simulink model "pendcart"  (R2015b)
settings: Solver=ode45  StartTime=0.0  StopTime=tsim  RelTol=1e-3
values from neighbouring files (symbols this model uses):
  b = 0.01    [old.m]
  c = 0.05    [old.m]
  g = 9.82    [old.m]
  K1 = -119.0071    [old.m]
  K2 = 0.0402    [old.m]
  l = 0.5    [old.m]
  M = 1    [old.m]
  m = 0.5    [old.m]
  p = 5.4277    [old.m]
  p1 = 25.4277    [old.m]
  theta0 = 5*pi/180    (= 0.0872664625997)    [old.m]
settings Model: Creator=Chris  LastModifiedBy=C3204612
settings DataIOCC: SaveFormat=Array  SignalLoggingSaveFormat=ModelDataLogs
settings OptimizationCC: ExpressionDepthLimit=2147483647  InitFltsAndDblsToZero=on
settings DebuggingCC: AlgebraicLoopMsg=none  SaveWithParameterizedLinksMsg=none  UnderspecifiedInitializationDetection=Classic  MergeDetectMultiDrivingBlocksExec=none  FcnCallInpInsideContextMsg=UseLocalSettings  StateNameClashWarn=warning
settings HardwareCC: ProdBitPerPointer=32  ProdLargestAtomicFloat=None  ProdIntDivRoundTo=Undefined  ProdEndianess=Unspecified  ProdWordSize=32  ProdHWDeviceType=32-bit Generic
settings GRTTargetCC: TargetFcnLib=ansi_tfl_tmw.mat  GeneratePreprocessorConditionals=Disable all  CombineOutputUpdateFcns=off  GRTInterface=on
settings ConfigComp: CovModelRefEnable=Off

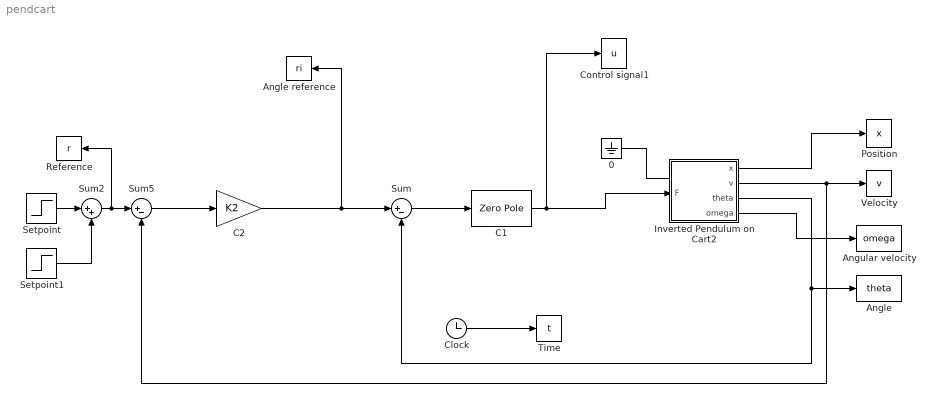
== system pendcart ==
  0 : Ground
  Angle : ToWorkspace  VariableName=theta  SampleTime=-1
  Angle reference : ToWorkspace  VariableName=ri  SampleTime=-1
  Angular velocity : ToWorkspace  VariableName=omega  SampleTime=-1
  C1 : ZeroPole  Zeros=[-p]  Poles=[-p1]  Gain=[K1]
  C2 : Gain  Gain=K2
  Clock : Clock
  Control signal1 : ToWorkspace  VariableName=u  SampleTime=-1
  Inverted Pendulum on Cart2 : Subsystem
  Position : ToWorkspace  VariableName=x  SampleTime=-1
  Reference : ToWorkspace  VariableName=r  SampleTime=-1
  Setpoint : Step  Time=10  After=0.5  SampleTime=0
  Setpoint1 : Step  Time=20  After=-0.5  SampleTime=0
  Sum : Sum  Inputs=|+-
  Sum2 : Sum  Inputs=|++
  Sum5 : Sum  Inputs=|+-
  Time : ToWorkspace  VariableName=t  SampleTime=-1
  Velocity : ToWorkspace  VariableName=v  SampleTime=-1
  wires:
  Clock/1 -> Time/1
  Inverted Pendulum on Cart2/1(x) -> Position/1
  Sum/1 -> C1/1
  C1/1 -> Control signal1/1, Inverted Pendulum on Cart2/1(F)
  Inverted Pendulum on Cart2/4(omega) -> Angular velocity/1
  Inverted Pendulum on Cart2/2(v) -> Velocity/1, Sum5/2
  Inverted Pendulum on Cart2/3(theta) -> Angle/1, Sum/2
  Sum5/1 -> C2/1
  C2/1 -> Angle reference/1, Sum/1
  Setpoint/1 -> Sum2/1
  Setpoint1/1 -> Sum2/2
  Sum2/1 -> Sum5/1, Reference/1
  0/1 -> ?

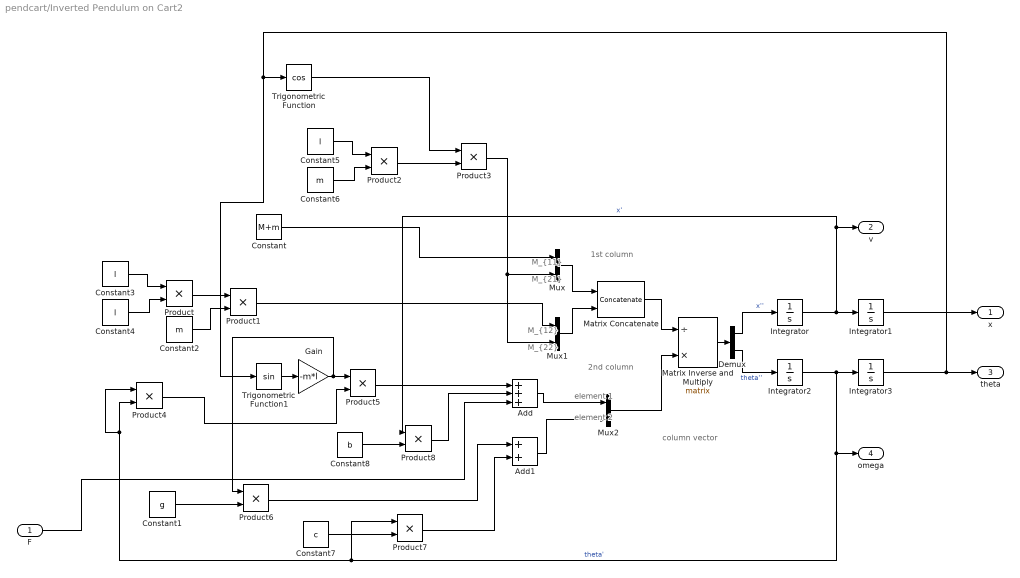
== system pendcart/Inverted Pendulum on Cart2 ==
  note: element 1
  note: M_{11}
  note: M_{21}
  note: M_{12}
  note: M_{22}
  note: 1st column
  note: 2nd column
  note: column vector
  note: element 2
  F : Inport
  Add : Sum  Inputs=+++
  Add1 : Sum
  Constant : Constant  Value=M+m
  Constant1 : Constant  Value=g
  Constant2 : Constant  Value=m
  Constant3 : Constant  Value=l
  Constant4 : Constant  Value=l
  Constant5 : Constant  Value=l
  Constant6 : Constant  Value=m
  Constant7 : Constant  Value=c
  Constant8 : Constant  Value=b
  Demux : Demux  Outputs=2
  Gain : Gain  Gain=-m*l
  Integrator : Integrator
  Integrator1 : Integrator
  Integrator2 : Integrator
  Integrator3 : Integrator  InitialCondition=theta0
  Matrix Concatenate : Concatenate  Mode=Multidimensional array  ConcatenateDimension=2
  Matrix Inverse and Multiply : Product  Inputs=/*  Multiplication=Matrix(*)
  Mux : Mux  Inputs=2
  Mux1 : Mux  Inputs=2
  Mux2 : Mux  Inputs=2
  Product{,1..8} (9 alike) : Product
  Trigonometric Function : Trigonometry  Operator=cos
  Trigonometric Function1 : Trigonometry
  x : Outport
  v : Outport  Port=2
  theta : Outport  Port=3
  omega : Outport  Port=4
  wires:
  Demux/1 -> Integrator/1  "x''"
  Integrator/1 -> Integrator1/1, Product8/1, v/1  "x'"
  Demux/2 -> Integrator2/1  "theta''"
  Integrator2/1 -> Integrator3/1, Product7/1, Product4/1, Product4/2, omega/1  "theta'"
  Matrix Inverse and Multiply/1 -> Demux/1
  Mux1/1 -> Matrix Concatenate/2
  Mux/1 -> Matrix Concatenate/1
  Matrix Concatenate/1 -> Matrix Inverse and Multiply/1
  Mux2/1 -> Matrix Inverse and Multiply/2
  Integrator1/1 -> x/1
  Integrator3/1 -> Trigonometric Function1/1, Trigonometric Function/1, theta/1
  Constant/1 -> Mux/1
  Constant2/1 -> Product1/2
  Product/1 -> Product1/1
  Constant3/1 -> Product/1
  Constant4/1 -> Product/2
  Product1/1 -> Mux1/1
  Constant5/1 -> Product2/1
  Constant6/1 -> Product2/2
  Product3/1 -> Mux1/2, Mux/2
  Product2/1 -> Product3/2
  Trigonometric Function/1 -> Product3/1
  Add/1 -> Mux2/1
  Add1/1 -> Mux2/2
  Trigonometric Function1/1 -> Gain/1
  Gain/1 -> Product6/1, Product5/1
  Product4/1 -> Product5/2
  Product5/1 -> Add/1
  Constant1/1 -> Product6/2
  Product6/1 -> Add1/1
  Constant7/1 -> Product7/2
  Product7/1 -> Add1/2
  F/1 -> Add/3
  Constant8/1 -> Product8/2
  Product8/1 -> Add/2
